simulink model "simu_lwr_rig_essentiels"  (Simulink 8.1)
settings: Solver=ode45  StartTime=0.0  StopTime=10.0  RelTol=1e-3
values from neighbouring files (symbols this model uses):
  fc1 = 11.9    [prog_princi_simu.m]
  fc2 = 11.5    [prog_princi_simu.m]
  fc3 = 8.98    [prog_princi_simu.m]
  fc4 = 8.35    [prog_princi_simu.m]
  fc5 = 8.31    [prog_princi_simu.m]
  fc6 = 4.72    [prog_princi_simu.m]
  fc7 = 6.04    [prog_princi_simu.m]
  fv1 = 14.4    [prog_princi_simu.m]
  fv2 = 15.3    [prog_princi_simu.m]
  fv3 = 6.55    [prog_princi_simu.m]
  fv4 = 11.0    (= 11)    [prog_princi_simu.m]
  fv5 = 4.29    [prog_princi_simu.m]
  fv6 = 2.26    [prog_princi_simu.m]
  fv7 = 1.6    [prog_princi_simu.m]
  g3 = -9.81    [prog_princi_simu.m]
  ia3 = 2.01    [prog_princi_simu.m]
  ia4 = 1.92    [prog_princi_simu.m]
  ia5 = 0.776    [prog_princi_simu.m]
  ia6 = 0.391    [prog_princi_simu.m]
  ia7 = 0.399    [prog_princi_simu.m]
  kd = 3.*w_cmd.*inerties-fv    [prog_princi_simu.m]
  ki = w_cmd.*w_cmd.*w_cmd.*inerties    [prog_princi_simu.m]
  kp = 3.*w_cmd.*w_cmd.*inerties    [prog_princi_simu.m]
  my2 = 3.3    [prog_princi_simu.m]
  my4 = -1.37    [prog_princi_simu.m]
  my5 = 0.049    [prog_princi_simu.m]
  my6 = 0.042    [prog_princi_simu.m]
  q0 = zeros(1,7)'    [prog_princi_simu.m]
  qd0 = zeros(1,7)'    [prog_princi_simu.m]
  rl3 = 0.400    (= 0.4)    [prog_princi_simu.m]
  rl5 = 0.390    (= 0.39)    [prog_princi_simu.m]
  tec = t(2)-t(1)    [prog_princi_simu.m]
  xx2 = 1.31    [prog_princi_simu.m]
  xx4 = 0.368    [prog_princi_simu.m]
  zz1 = 3.20    (= 3.2)    [prog_princi_simu.m]
  zz2 = 4.46    [prog_princi_simu.m]
  zz4 = 0.491    [prog_princi_simu.m]
undefined symbols (not defined in the file or in its folder): DiscIntNeverNeededParam
settings Model: Creator=maxime  LastModifiedBy=adminuser
settings DebuggingCC: StrictBusMsg=Warning
settings RTWCC: TargetLang=C++  RTWCompilerOptimization=On

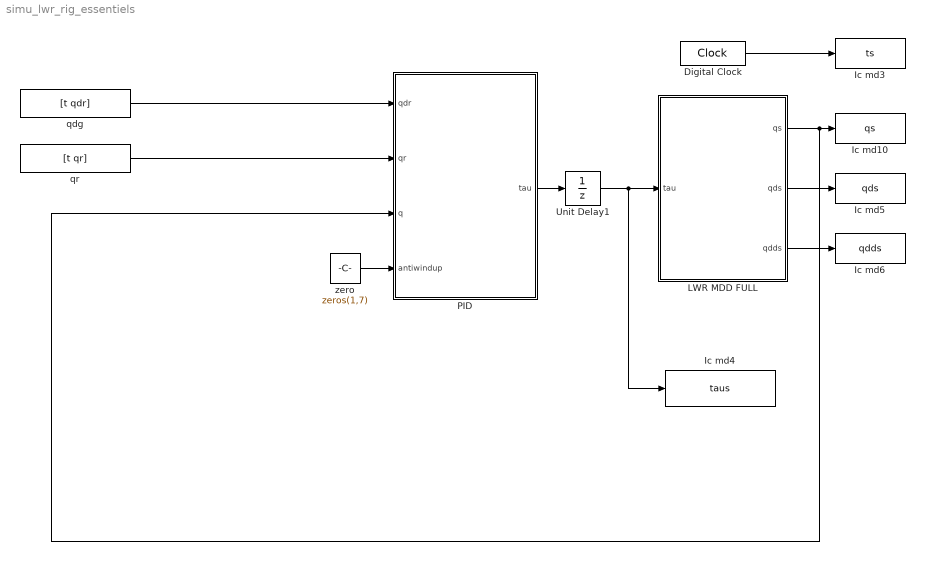
== system simu_lwr_rig_essentiels ==
  Digital Clock : DigitalClock  SampleTime=tec
  Ic md10 : ToWorkspace  VariableName=qs  SampleTime=tec
  Ic md3 : ToWorkspace  VariableName=ts  SampleTime=tec
  Ic md4 : ToWorkspace  VariableName=taus  SampleTime=tec
  Ic md5 : ToWorkspace  VariableName=qds  SampleTime=tec
  Ic md6 : ToWorkspace  VariableName=qdds  SampleTime=tec
  LWR MDD FULL : Subsystem
  "PID " : Subsystem
  Unit Delay1 : UnitDelay  InitialCondition=[ 0 0 0 0 0 0 0 ]  SampleTime=tec
  qdg : FromWorkspace  VariableName=[t qdr]  SampleTime=tec
  qr : FromWorkspace  VariableName=[t qr]  SampleTime=tec
  zero : Constant  Value=zeros(1,7)  SampleTime=Inf
  wires:
  Digital Clock/1 -> Ic md3/1
  LWR MDD FULL/2(qds) -> Ic md5/1
  LWR MDD FULL/3(qdds) -> Ic md6/1
  Unit Delay1/1 -> Ic md4/1, LWR MDD FULL/1(tau)
  qdg/1 -> "PID "/1(qdr)
  LWR MDD FULL/1(qs) -> Ic md10/1, "PID "/3(q)
  qr/1 -> "PID "/2(qr)
  zero/1 -> "PID "/4(antiwindup)
  "PID "/1(tau) -> Unit Delay1/1

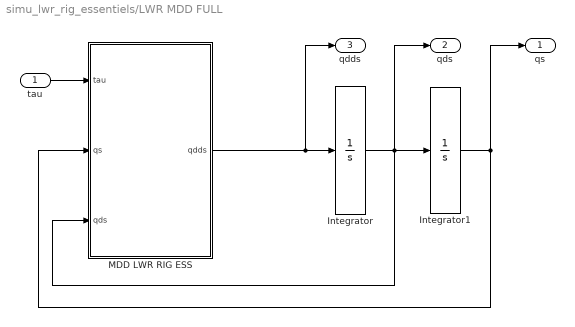
== system simu_lwr_rig_essentiels/LWR MDD FULL ==
  tau : Inport
  Integrator : Integrator  InitialCondition=qd0  ZeroCross=off
  Integrator1 : Integrator  InitialCondition=q0  ZeroCross=off
  MDD LWR RIG ESS : MATLAB Function  TreatAsAtomicUnit=on
  qs : Outport
  qds : Outport  Port=2
  qdds : Outport  Port=3
  wires:
  Integrator/1 -> qds/1, MDD LWR RIG ESS/3(qds), Integrator1/1
  Integrator1/1 -> MDD LWR RIG ESS/2(qs), qs/1
  tau/1 -> MDD LWR RIG ESS/1(tau)
  MDD LWR RIG ESS/1(qdds) -> Integrator/1, qdds/1

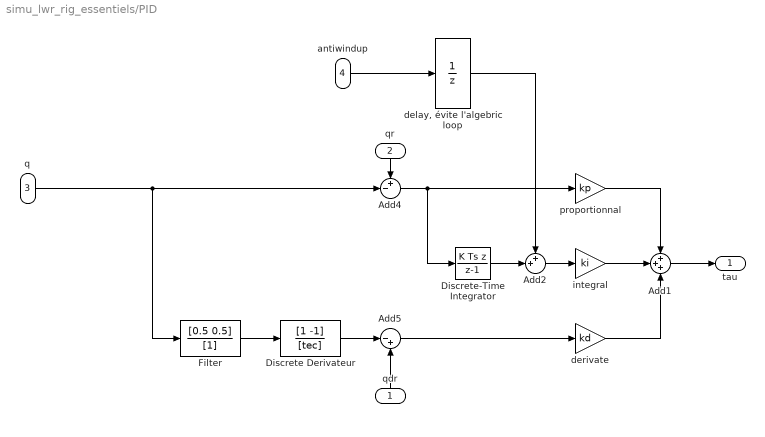
== system simu_lwr_rig_essentiels/PID  ==
  qdr : Inport
  qr : Inport  Port=2
  q : Inport  Port=3
  antiwindup : Inport  Port=4
  " Filter" : DiscreteFilter  Numerator=[0.5 0.5]  Denominator=[1]  SampleTime=tec
  Add1 : Sum  Inputs=+++
  Add2 : Sum  Inputs=++|
  Add4 : Sum  Inputs=+-|
  Add5 : Sum  Inputs=|-+
  Discrete Derivateur : DiscreteFilter  Numerator=[1 -1]  Denominator=[tec]  SampleTime=tec
  Discrete-Time Integrator : DiscreteIntegrator  IntegratorMethod=Integration: Backward Euler  SampleTime=tec  ICPrevOutput=DiscIntNeverNeededParam  ICPrevScaledInput=DiscIntNeverNeededParam
  "delay, évite l'algebric loop" : UnitDelay  InitialCondition=[ 0 0 0 0 0 0 0 ]  SampleTime=tec
  derivate : Gain  Gain=kd
  integral : Gain  Gain=ki
  proportionnal : Gain  Gain=kp
  tau : Outport
  wires:
  proportionnal/1 -> Add1/1
  Add1/1 -> tau/1
  q/1 -> " Filter"/1, Add4/2
  Add4/1 -> Discrete-Time Integrator/1, proportionnal/1
  " Filter"/1 -> Discrete Derivateur/1
  derivate/1 -> Add1/3
  Discrete Derivateur/1 -> Add5/1
  integral/1 -> Add1/2
  Add5/1 -> derivate/1
  qdr/1 -> Add5/2
  qr/1 -> Add4/1
  Add2/1 -> integral/1
  Discrete-Time Integrator/1 -> Add2/2
  "delay, évite l'algebric loop"/1 -> Add2/1
  antiwindup/1 -> "delay, évite l'algebric loop"/1

== matlab function LWR MDD FULL/MDD LWR RIG ESS ==
  data: tau input double size=7; qs input double size=7; qds input double size=7; rl3 parameter double size=1; rl5 parameter double size=1; g3 parameter double size=1; qdds output double size=7; fv1 parameter double size=1; fc1 parameter double size=1; fv2 parameter double size=1; fc2 parameter double size=1; ia3 parameter double size=1; fv3 parameter double size=1; fc3 parameter double size=1; ia4 parameter double size=1; fv4 parameter double size=1; fc4 parameter double size=1; ia5 parameter double size=1; fv5 parameter double size=1; fc5 parameter double size=1; ia6 parameter double size=1; fv6 parameter double size=1; fc6 parameter double size=1; ia7 parameter double size=1; fv7 parameter double size=1; fc7 parameter double size=1; zz1 parameter double size=1; xx2 parameter double size=1; zz2 parameter double size=1; my2 parameter double size=1; xx4 parameter double size=1; zz4 parameter double size=1; my4 parameter double size=1; my5 parameter double size=1; my6 parameter double size=1
%    lwr 4+ irccyn (version rigide -paramètres essentiels seulements-)
%    copyright (c) 2014 by irccyn, anthony jubien (anthony.jubien@irccyn.ec-nantes.fr)
%    creation: 1.0  date: 18/11/14   anthony jubien
%    revision: 	    date: 18/11/14   anthony jubien
%    nécessite la toolbox matlab coder et visual studio pour convertir en .c/.mex function
%    !!divulgation/distribution sans l'accord de l'auteur prohibée!!

function qdds = lwr_mdd_rig_ess(tau, qs, qds, rl3 , rl5 , g3 , fv1,fc1,fv2,fc2,ia3,fv3,fc3,ia4,fv4,fc4,ia5,fv5,fc5,ia6,fv6,fc6,ia7,fv7,fc7,zz1,xx2,zz2,my2,xx4,zz4,my4,my5,my6)

d2spi = 0.63661977236758134307553505349006 ; % = 2/pi
ta = 100 ; 
% sign(X) remplacé par d2spi*atan(ta*(X) pour éviter les instabilités numériques du passage par 0

%positions
q1   = qs(1) ;
q2   = qs(2) ;
q3   = qs(3) ;
q4   = qs(4) ;
q5   = qs(5) ;
q6   = qs(6) ;
q7   = qs(7) ;

%vitesses
qd1   = qds(1) ;
qd2   = qds(2) ;
qd3   = qds(3) ;
qd4   = qds(4) ;
qd5   = qds(5) ;
qd6   = qds(6) ;
qd7   = qds(7) ;

%couples moteurs
gam1   = tau(1) ;
gam2   = tau(2) ;
gam3   = tau(3) ;
gam4   = tau(4) ;
gam5   = tau(5) ;
gam6   = tau(6) ;
gam7   = tau(7) ;

% modèle dynamique direct du kuka lwr (paramètres essentiels seulements)
% calculés par symoro+

s2=sin(q2);
c2=cos(q2);
s3=sin(q3);
c3=cos(q3);
s4=sin(q4);
c4=cos(q4);
s5=sin(q5);
c5=cos(q5);
s6=sin(q6);
c6=cos(q6);
wi12=qd1.*s2;
wi22=c2.*qd1;
wi13=-(qd2.*s3) + c3.*wi12;
wi23=-(c3.*qd2) - s3.*wi12;
w33=qd3 + wi22;
jpr113=-(rl3.*s3);
jpr133=-(c3.*rl3);
jpr213=-(c3.*rl3);
jpr233=rl3.*s3;
wi14=-(s4.*w33) + c4.*wi13;
wi24=-(c4.*w33) - s4.*wi13;
w34=qd4 + wi23;
wi15=s5.*w34 + c5.*wi14;
wi25=c5.*w34 - s5.*wi14;
w35=qd5 - wi24;
jpr115=-(rl5.*s5);
jpr135=c5.*rl5;
jpr215=-(c5.*rl5);
jpr235=-(rl5.*s5);
wi16=s6.*w35 + c6.*wi15;
wi26=c6.*w35 - s6.*wi15;
w36=qd6 - wi25;
jw12=wi12.*xx2;
jw32=qd2.*zz2;
kw12=jw32.*wi22;
kw22=jw12.*qd2 - jw32.*wi12;
kw32=-(jw12.*wi22);
wq12=qd2.*wi22;
wq22=-(qd2.*wi12);
wq13=qd3.*wi23;
wq23=-(qd3.*wi13);
lw13=-(qd2.*rl3.*s3.*wi22) + c3.*rl3.*wi12.*wi22;
lw23=-(c3.*qd2.*rl3.*wi22) - rl3.*s3.*wi12.*wi22;
lw33=-(qd2.^2.*rl3) - rl3.*wi12.^2;
jw14=wi14.*xx4;
jw34=w34.*zz4;
kw14=jw34.*wi24;
kw24=jw14.*w34 - jw34.*wi14;
kw34=-(jw14.*wi24);
sw14=my4.*wi14.*wi24;
sw24=-(my4.*w34.^2) - my4.*wi14.^2;
sw34=my4.*w34.*wi24;
wq14=qd4.*wi24;
wq24=-(qd4.*wi14);
sw15=my5.*wi15.*wi25;
sw25=-(my5.*w35.^2) - my5.*wi15.^2;
sw35=my5.*w35.*wi25;
wq15=qd5.*wi25;
wq25=-(qd5.*wi15);
lw15=-(rl5.*s5.*w34.*wi24) - c5.*rl5.*wi14.*wi24;
lw25=-(c5.*rl5.*w34.*wi24) + rl5.*s5.*wi14.*wi24;
lw35=-(rl5.*w34.^2) - rl5.*wi14.^2;
sw16=my6.*wi16.*wi26;
sw26=-(my6.*w36.^2) - my6.*wi16.^2;
sw36=my6.*w36.*wi26;
wq16=qd6.*wi26;
jd7=1./ia7;
gw7=gam7 - fv7.*qd7 - fc7.*d2spi*atan(ta*(qd7));
jd6=1./ia6;
ju46=-(jd6.*my6);
gw6=gam6 - fv6.*qd6 - fc6.*d2spi*atan(ta*(qd6));
gk446=ju46.*my6;
ng66=my6.*wq16;
vs46=gw6.*ju46;
ap46=sw16 + vs46;
ap66=ng66 + sw36;
gx436=-(c6.*my6);
gx446=c6.*gk446;
gx636=-(my6.*s6);
gx646=gk446.*s6;
tkt516=-(c6.*my6);
tkt536=-(my6.*s6);
tkt446=c6.*gx446;
tkt646=c6.*gx646;
tkt666=gx646.*s6;
vbe45=-(ap46.*c6) - sw15 + s6.*sw26;
vbe55=ap66 - sw25;
vbe65=-(ap46.*s6) - c6.*sw26 - sw35;
jd5=1./ia5;
ju45=-(jd5.*my5);
ju55=jd5.*tkt536;
gw5=gam5 - fv5.*qd5 - fc5.*d2spi*atan(ta*(qd5));
gk445=ju45.*my5 + tkt446;
gk455=-(ju45.*tkt536);
gk545=ju55.*my5;
gk555=-(ju55.*tkt536);
ng15=lw35.*my5 + lw25.*tkt516;
ng25=-(gx436.*lw15) - gx636.*lw35;
ng35=-(lw15.*my5) + lw25.*tkt536;
ng45=gk445.*lw15 + gk455.*lw25 + lw35.*tkt646 - gx436.*wq25;
ng55=gk545.*lw15 + gk555.*lw25 + tkt516.*wq15;
ng65=lw15.*tkt646 + lw35.*tkt666 + my5.*wq15 - gx636.*wq25;
vs45=gw5.*ju45 + ng45;
vs55=gw5.*ju55 + ng55;
ap45=-vbe45 + vs45;
ap55=-vbe55 + vs55;
ap65=ng65 - vbe65;
gx115=jpr215.*tkt516;
gx125=-(gx436.*jpr115);
gx145=gk445.*jpr115 + gk545.*jpr215 + gx436.*s5;
gx155=gk455.*jpr115 + gk555.*jpr215 + c5.*tkt516;
gx315=jpr235.*tkt516;
gx325=-(gx436.*jpr135);
gx335=-(jpr135.*my5) + jpr235.*tkt536;
gx345=-(c5.*gx436) + gk445.*jpr135 + gk545.*jpr235;
gx355=gk455.*jpr135 + gk555.*jpr235 + s5.*tkt516;
gx415=-(s5.*tkt516);
gx425=-(c5.*gx436);
gx435=-(c5.*my5) - s5.*tkt536;
gx445=c5.*gk445 - gk545.*s5;
gx455=c5.*gk455 - gk555.*s5;
gx615=c5.*tkt516;
gx625=-(gx436.*s5);
gx635=-(my5.*s5) + c5.*tkt536;
gx645=c5.*gk545 + gk445.*s5;
gx655=c5.*gk555 + gk455.*s5;
gx665=s5.*tkt646;
tkt115=c5.*gx115 + gx145.*jpr115 + gx155.*jpr215 - gx125.*s5;
tkt215=jpr115.*my5 - jpr215.*tkt536;
tkt315=c5.*gx315 + gx345.*jpr115 + gx355.*jpr215 - gx325.*s5;
tkt415=c5.*gx415 + gx445.*jpr115 + gx455.*jpr215 - gx425.*s5;
tkt515=-(c5.*my5) - gx636.*s5 - jpr115.*tkt646;
tkt615=c5.*gx615 + gx645.*jpr115 + gx655.*jpr215 - gx625.*s5;
tkt335=c5.*gx325 + gx345.*jpr135 + gx355.*jpr235 + gx315.*s5;
tkt435=c5.*gx425 + gx445.*jpr135 + gx455.*jpr235 + gx415.*s5;
tkt535=c5.*gx636 - my5.*s5 - jpr135.*tkt646;
tkt635=c5.*gx625 + gx645.*jpr135 + gx655.*jpr235 + gx615.*s5;
tkt445=c5.*gx445 - gx455.*s5;
tkt545=-(c5.*tkt646);
tkt645=c5.*gx645 - gx655.*s5;
tkt665=c5.*gx655 + gx645.*s5;
mje114=tkt115 + xx4;
mje614=my4 + tkt615;
mje334=tkt335 + zz4;
mje434=-my4 + tkt435;
vbe14=-(ap45.*jpr115) - ap55.*jpr215 - kw14 - c5.*ng15 + ng25.*s5;
vbe24=-kw24 + ng35;
vbe34=-(ap45.*jpr135) - ap55.*jpr235 - kw34 - c5.*ng25 - ng15.*s5;
vbe44=-(ap45.*c5) + ap55.*s5 - sw14;
vbe54=ap65 - sw24;
vbe64=-(ap55.*c5) - ap45.*s5 - sw34;
jd4=1./(ia4 + mje334);
ju14=jd4.*tkt315;
ju24=-(gx335.*jd4);
ju34=jd4.*mje334;
ju44=jd4.*mje434;
ju54=jd4.*tkt535;
ju64=jd4.*tkt635;
gw4=gam4 - fv4.*qd4 + vbe34 - fc4.*d2spi*atan(ta*(qd4));
gk114=mje114 - ju14.*tkt315;
gk124=gx335.*ju14 + tkt215;
gk134=-(ju14.*mje334) + tkt315;
gk214=tkt215 - ju24.*tkt315;
gk224=gx335.*ju24;
gk234=-gx335 - ju24.*mje334;
gk314=tkt315 - ju34.*tkt315;
gk324=-gx335 + gx335.*ju34;
gk334=mje334 - ju34.*mje334;
gk414=-(ju44.*tkt315) + tkt415;
gk424=-gx435 + gx335.*ju44;
gk434=-(ju44.*mje334) + mje434;
gk444=-(ju44.*mje434) + tkt445;
gk454=-(ju44.*tkt535) + tkt545;
gk464=-(ju44.*tkt635) + tkt645;
gk514=-(ju54.*tkt315) + tkt515;
gk524=gx335.*ju54;
gk534=-(ju54.*mje334) + tkt535;
gk544=-(ju54.*mje434) + tkt545;
gk554=-(ju54.*tkt535) + tkt666;
gk564=-gx665 - ju54.*tkt635;
gk614=mje614 - ju64.*tkt315;
gk624=-gx635 + gx335.*ju64;
gk634=-(ju64.*mje334) + tkt635;
gk644=-(ju64.*mje434) + tkt645;
gk654=-gx665 - ju64.*tkt535;
gk664=-(ju64.*tkt635) + tkt665;
ng14=gk114.*wq14 + gk124.*wq24;
ng24=gk214.*wq14 + gk224.*wq24;
ng34=gk314.*wq14 + gk324.*wq24;
ng44=gk414.*wq14 + gk424.*wq24;
ng54=gk514.*wq14 + gk524.*wq24;
ng64=gk614.*wq14 + gk624.*wq24;
vs14=gw4.*ju14 + ng14;
vs24=gw4.*ju24 + ng24;
vs34=gw4.*ju34 + ng34;
vs44=gw4.*ju44 + ng44;
vs54=gw4.*ju54 + ng54;
vs64=gw4.*ju64 + ng64;
ap14=-vbe14 + vs14;
ap24=-vbe24 + vs24;
ap34=-vbe34 + vs34;
ap44=-vbe44 + vs44;
ap54=-vbe54 + vs54;
ap64=-vbe64 + vs64;
gx114=c4.*gk114 - gk214.*s4;
gx124=c4.*gk124 - gk224.*s4;
gx314=-(c4.*gk214) - gk114.*s4;
gx324=-(c4.*gk224) - gk124.*s4;
gx334=-(c4.*gk234) - gk134.*s4;
gx414=c4.*gk414 - gk514.*s4;
gx424=c4.*gk424 - gk524.*s4;
gx434=c4.*gk434 - gk534.*s4;
gx444=c4.*gk444 - gk544.*s4;
gx454=c4.*gk454 - gk554.*s4;
gx614=-(c4.*gk514) - gk414.*s4;
gx624=-(c4.*gk524) - gk424.*s4;
gx634=-(c4.*gk534) - gk434.*s4;
gx644=-(c4.*gk544) - gk444.*s4;
gx654=-(c4.*gk554) - gk454.*s4;
gx664=-(c4.*gk564) - gk464.*s4;
tkt114=c4.*gx114 - gx124.*s4;
tkt214=c4.*gk314 - gk324.*s4;
tkt314=c4.*gx314 - gx324.*s4;
tkt414=c4.*gx414 - gx424.*s4;
tkt514=c4.*gk614 - gk624.*s4;
tkt614=c4.*gx614 - gx624.*s4;
tkt334=-(c4.*gx324) - gx314.*s4;
tkt434=-(c4.*gx424) - gx414.*s4;
tkt534=-(c4.*gk624) - gk614.*s4;
tkt634=-(c4.*gx624) - gx614.*s4;
tkt444=c4.*gx444 - gx454.*s4;
tkt544=c4.*gk644 - gk654.*s4;
tkt644=c4.*gx644 - gx654.*s4;
vbe13=-(ap14.*c4) + ap24.*s4;
vbe33=ap24.*c4 + ap14.*s4;
vbe43=-(ap44.*c4) + ap54.*s4;
jd3=1./(ia3 + tkt334);
ju13=jd3.*tkt314;
ju23=gx334.*jd3;
ju33=jd3.*tkt334;
ju43=jd3.*tkt434;
ju53=jd3.*tkt534;
ju63=jd3.*tkt634;
gw3=gam3 - fv3.*qd3 + vbe33 - fc3.*d2spi*atan(ta*(qd3));
gk113=tkt114 - ju13.*tkt314;
gk123=-(gx334.*ju13) + tkt214;
gk133=tkt314 - ju13.*tkt334;
gk143=tkt414 - ju13.*tkt434;
gk153=tkt514 - ju13.*tkt534;
gk163=tkt614 - ju13.*tkt634;
gk213=tkt214 - ju23.*tkt314;
gk223=gk334 - gx334.*ju23;
gk233=gx334 - ju23.*tkt334;
gk243=gx434 - ju23.*tkt434;
gk253=gk634 - ju23.*tkt534;
gk263=gx634 - ju23.*tkt634;
gk313=tkt314 - ju33.*tkt314;
gk323=gx334 - gx334.*ju33;
gk333=tkt334 - ju33.*tkt334;
gk343=tkt434 - ju33.*tkt434;
gk353=tkt534 - ju33.*tkt534;
gk363=tkt634 - ju33.*tkt634;
gk413=-(ju43.*tkt314) + tkt414;
gk423=gx434 - gx334.*ju43;
gk433=-(ju43.*tkt334) + tkt434;
gk443=-(ju43.*tkt434) + tkt444;
gk453=-(ju43.*tkt534) + tkt544;
gk463=-(ju43.*tkt634) + tkt644;
gk513=-(ju53.*tkt314) + tkt514;
gk523=gk634 - gx334.*ju53;
gk533=-(ju53.*tkt334) + tkt534;
gk543=-(ju53.*tkt434) + tkt544;
gk553=gk664 - ju53.*tkt534;
gk563=gx664 - ju53.*tkt634;
gk613=-(ju63.*tkt314) + tkt614;
gk623=gx634 - gx334.*ju63;
gk633=-(ju63.*tkt334) + tkt634;
gk643=-(ju63.*tkt434) + tkt644;
gk653=gx664 - ju63.*tkt534;
ng13=gk143.*lw13 + gk153.*lw23 + gk163.*lw33 + gk113.*wq13 + gk123.*wq23;
ng23=gk243.*lw13 + gk253.*lw23 + gk263.*lw33 + gk213.*wq13 + gk223.*wq23;
ng33=gk343.*lw13 + gk353.*lw23 + gk363.*lw33 + gk313.*wq13 + gk323.*wq23;
ng43=gk443.*lw13 + gk453.*lw23 + gk463.*lw33 + gk413.*wq13 + gk423.*wq23;
ng53=gk543.*lw13 + gk553.*lw23 + gk563.*lw33 + gk513.*wq13 + gk523.*wq23;
vs13=gw3.*ju13 + ng13;
vs23=gw3.*ju23 + ng23;
vs33=gw3.*ju33 + ng33;
vs43=gw3.*ju43 + ng43;
vs53=gw3.*ju53 + ng53;
ap13=-vbe13 + vs13;
ap23=ap34 + vs23;
ap33=-vbe33 + vs33;
ap43=-vbe43 + vs43;
ap53=ap64 + vs53;
gx113=c3.*gk113 + gk413.*jpr113 + gk513.*jpr213 - gk213.*s3;
gx123=c3.*gk123 + gk423.*jpr113 + gk523.*jpr213 - gk223.*s3;
gx143=c3.*gk143 + gk443.*jpr113 + gk543.*jpr213 - gk243.*s3;
gx153=c3.*gk153 + gk453.*jpr113 + gk553.*jpr213 - gk253.*s3;
gx313=-(c3.*gk213) + gk413.*jpr133 + gk513.*jpr233 - gk113.*s3;
gx323=-(c3.*gk223) + gk423.*jpr133 + gk523.*jpr233 - gk123.*s3;
gx333=-(c3.*gk233) + gk433.*jpr133 + gk533.*jpr233 - gk133.*s3;
gx343=-(c3.*gk243) + gk443.*jpr133 + gk543.*jpr233 - gk143.*s3;
gx353=-(c3.*gk253) + gk453.*jpr133 + gk553.*jpr233 - gk153.*s3;
gx413=c3.*gk413 - gk513.*s3;
gx423=c3.*gk423 - gk523.*s3;
gx433=c3.*gk433 - gk533.*s3;
gx443=c3.*gk443 - gk543.*s3;
gx453=c3.*gk453 - gk553.*s3;
tkt113=c3.*gx113 + gx143.*jpr113 + gx153.*jpr213 - gx123.*s3;
tkt213=c3.*gk313 + gk343.*jpr113 + gk353.*jpr213 - gk323.*s3;
tkt313=c3.*gx313 + gx343.*jpr113 + gx353.*jpr213 - gx323.*s3;
tkt413=c3.*gx413 + gx443.*jpr113 + gx453.*jpr213 - gx423.*s3;
tkt513=c3.*gk613 + gk643.*jpr113 + gk653.*jpr213 - gk623.*s3;
tkt333=-(c3.*gx323) + gx343.*jpr133 + gx353.*jpr233 - gx313.*s3;
tkt433=-(c3.*gx423) + gx443.*jpr133 + gx453.*jpr233 - gx413.*s3;
tkt533=-(c3.*gk623) + gk643.*jpr133 + gk653.*jpr233 - gk613.*s3;
mje112=tkt113 + xx2;
mje332=tkt333 + zz2;
mje432=-my2 + tkt433;
vbe12=-(ap13.*c3) - ap43.*jpr113 - ap53.*jpr213 - kw12 + ap23.*s3;
vbe22=-ap33 - kw22;
vbe32=ap23.*c3 - ap43.*jpr133 - ap53.*jpr233 - kw32 + ap13.*s3;
jd2=1./mje332;
ju12=jd2.*tkt313;
ju22=gx333.*jd2;
ju42=jd2.*mje432;
ju52=jd2.*tkt533;
gw2=gam2 - fv2.*qd2 + vbe32 - fc2.*d2spi*atan(ta*(qd2));
gk112=mje112 - ju12.*tkt313;
gk122=-(gx333.*ju12) + tkt213;
gk212=tkt213 - ju22.*tkt313;
gk222=gk333 - gx333.*ju22;
gk412=-(ju42.*tkt313) + tkt413;
gk422=gx433 - gx333.*ju42;
gk512=-(ju52.*tkt313) + tkt513;
gk522=gk633 - gx333.*ju52;
ng12=gk112.*wq12 + gk122.*wq22;
ng22=gk212.*wq12 + gk222.*wq22;
vs12=gw2.*ju12 + ng12;
vs22=gw2.*ju22 + ng22;
ap12=-vbe12 + vs12;
ap22=-vbe22 + vs22;
gx312=c2.*gk212 + gk112.*s2;
gx322=c2.*gk222 + gk122.*s2;
gx612=c2.*gk512 + gk412.*s2;
gx622=c2.*gk522 + gk422.*s2;
tkt332=c2.*gx322 + gx312.*s2;
tkt632=c2.*gx622 + gx612.*s2;
mje331=tkt332 + zz1;
vbe31=-(ap22.*c2) - ap12.*s2;
jd1=1./mje331;
ju61=jd1.*tkt632;
gw1=gam1 - fv1.*qd1 + vbe31 - fc1.*d2spi*atan(ta*(qd1));
gu1=-(g3.*ju61);
qdp1=-gu1 + gw1.*jd1;
vr12=qdp1.*s2 + wq12;
vr22=c2.*qdp1 + wq22;
vr42=-(g3.*s2);
vr52=-(c2.*g3);
gu2=ju12.*vr12 + ju22.*vr22 + ju42.*vr42 + ju52.*vr52;
qdp2=-gu2 + gw2.*jd2;
vr13=-(qdp2.*s3) + c3.*vr12 + wq13;
vr23=-(c3.*qdp2) - s3.*vr12 + wq23;
vr43=lw13 + jpr133.*qdp2 + jpr113.*vr12 + c3.*vr42;
vr53=lw23 + jpr233.*qdp2 + jpr213.*vr12 - s3.*vr42;
vr63=lw33 + vr52;
gu3=ju13.*vr13 + ju33.*vr22 + ju23.*vr23 + ju43.*vr43 + ju53.*vr53 + ju63.*vr63;
qdp3=-gu3 + gw3.*jd3;
wp33=qdp3 + vr22;
vr14=c4.*vr13 - s4.*wp33 + wq14;
vr24=-(s4.*vr13) - c4.*wp33 + wq24;
vr44=c4.*vr43 - s4.*vr63;
vr54=-(s4.*vr43) - c4.*vr63;
gu4=ju14.*vr14 + ju34.*vr23 + ju24.*vr24 + ju44.*vr44 + ju64.*vr53 + ju54.*vr54;
qdp4=-gu4 + gw4.*jd4;
wp34=qdp4 + vr23;
vr45=lw15 + jpr115.*vr14 + c5.*vr44 + s5.*vr53 + jpr135.*wp34;
vr55=lw25 + jpr215.*vr14 - s5.*vr44 + c5.*vr53 + jpr235.*wp34;
vr65=lw35 - vr54;
gu5=ju45.*vr45 + ju55.*vr55;
qdp5=-gu5 + gw5.*jd5;
vr46=c6.*vr45 + s6.*vr65;
gu6=ju46.*vr46;
qdp6=-gu6 + gw6.*jd6;
qdp7=gw7.*jd7;


qdds = [ qdp1 qdp2 qdp3 qdp4 qdp5 qdp6 qdp7 ]';

end
